simulink model "ME780_A3_Q3b"  (R2025b)
settings: Solver=FixedStepAuto  StartTime=0.0  StopTime=12  FixedStep=0.0005  RelTol=1e-3
libraries: Solver_SF x1, slpidlib x1
settings Model: Creator=r3anjum  LastModifiedBy=r3anjum

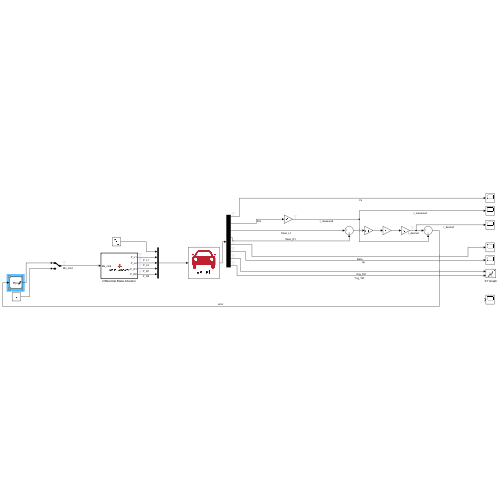
[thumbnail: Simulink's stored preview of the top-level diagram]
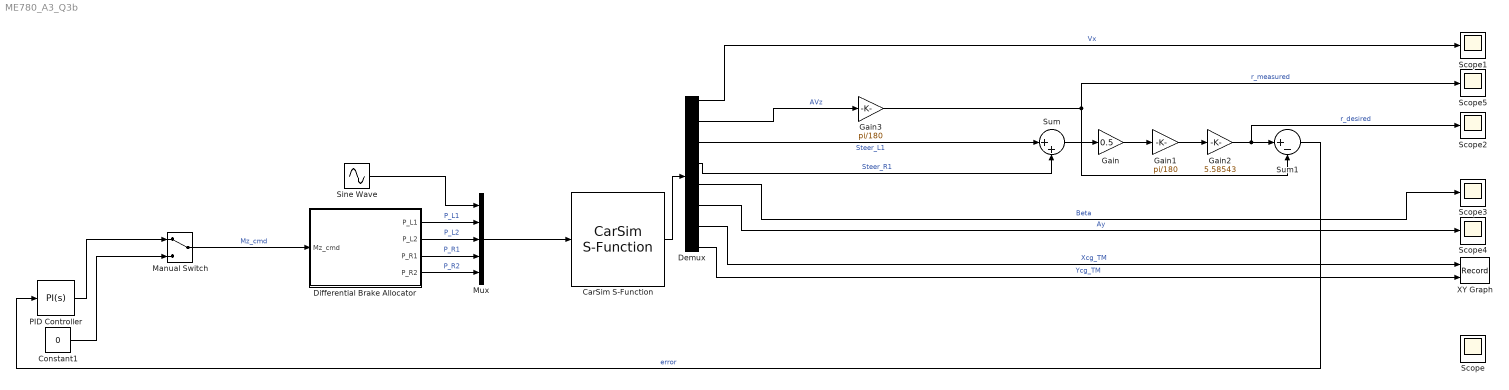
== system ME780_A3_Q3b ==
  CarSim S-Function : Solver_SF/CarSim S-Function  Priority=1  SIMFILE=simfile.sim  Run_RTs=off  vs_state_ind=Run  StopMode_ind=Vehicle Model
  Constant1 : Constant  Value=0
  Demux : Demux  Outputs=8
  Differential Brake Allocator : MATLAB Function  TreatAsAtomicUnit=on
  Gain : Gain  Gain=0.5
  Gain1 : Gain  Gain=pi/180
  Gain2 : Gain  Gain=5.58543
  Gain3 : Gain  Gain=pi/180
  Manual Switch : ManualSwitch
  Mux : Mux  Inputs=5
  PID Controller : slpidlib/PID Controller  Controller=PI  Form=Parallel  TimeDomain=Continuous-time  UseExternalTs=off  SampleTime=-1  IntegratorMethod=Forward Euler  FilterMethod=Forward Euler  ControllerParametersSource=internal  P=28835.61  I=57671.23  UseKiTs=off  D=0  UseExternalDerivativeSource=off  N=100  UseFilter=on  TunerSelectOption=Transfer Function Based (PID Tuner App)  InitialConditionSource=internal  InitialConditionForIntegrator=0  InitialConditionForFilter=0  DifferentiatorICPrevScaledInput=0  ExternalReset=none  TrackingMode=off  Kt=1  LimitOutput=on  SatLimitsSource=internal  UpperSaturationLimit=2800  LowerSaturationLimit=-2800  LinearizeAsGain=on  AntiWindupMode=clamping  Kb=1  LimitIntegrator=off  UpperIntegratorSaturationLimit=inf  LowerIntegratorSaturationLimit=-inf  POutMin=[]  POutMax=[]  IOutMin=[]  IOutMax=[]  DOutMin=[]  DOutMax=[]  NOutMin=[]  NOutMax=[]  SumOutMin=[]  SumOutMax=[]  SaturationOutMin=[]  SaturationOutMax=[]  PParamMin=[]  PParamMax=[]  IParamMin=[]  IParamMax=[]  DParamMin=[]  DParamMax=[]  NParamMin=[]  NParamMax=[]  KbParamMin=[]  KbParamMax=[]  KtParamMin=[]  KtParamMax=[]  KbOutMin=[]  KbOutMax=[]  KtOutMin=[]  KtOutMax=[]  IntegratorOutMin=[]  IntegratorOutMax=[]  FilterOutMin=[]  FilterOutMax=[]  SumI1OutMin=[]  SumI1OutMax=[]  SumI2OutMin=[]  SumI2OutMax=[]  SumI3OutMin=[]  SumI3OutMax=[]  SumI4OutMin=[]  SumI4OutMax=[]  SumDOutMin=[]  SumDOutMax=[]  DifferentiatorOutMin=[]  DifferentiatorOutMax=[]  FilterDiffOutCoefMin=[]  FilterDiffOutCoefMax=[]  ReciprocalOutMin=[]  ReciprocalOutMax=[]  SumDenOutMin=[]  SumDenOutMax=[]  SumNumOutMin=[]  SumNumOutMax=[]  DivideOutMin=[]  DivideOutMax=[]  UdiffTsProdOutMin=[]  UdiffTsProdOutMax=[]  NTsProdOutMin=[]  NTsProdOutMax=[]  UintegralTsProdOutMin=[]  UintegralTsProdOutMax=[]  UngainTsProdOutMin=[]  UngainTsProdOutMax=[]  ClampingZeroOutDataTypeStr=Inherit: Inherit via back propagation  ClampingZeroOutMin=[]  ClampingZeroOutMax=[]  FilterDenConstantOutDataTypeStr=Inherit: Inherit via back propagation  FilterDenConstantOutMin=[]  FilterDenConstantOutMax=[]  PCopyOutDataTypeStr=Inherit: Inherit via back propagation  PCopyOutMin=[]  PCopyOutMax=[]  NCopyOutDataTypeStr=Inherit: Inherit via back propagation  NCopyOutMin=[]  NCopyOutMax=[]  IntegratorContinuousStateAttributes=''  IntegratorStateMustResolveToSignalObject=off  IntegratorRTWStateStorageClass=Auto  FilterContinuousStateAttributes=''  FilterStateMustResolveToSignalObject=off  FilterRTWStateStorageClass=Auto  ParallelPVariant=InternalParameters  IdealPVariant=Disabled  IVariant=InternalParameters  DVariant=Disabled  IntegratorVariant=Continuous  SatVariant=Enabled  AWVariant=ContClampingParallel  PCopyVariant=Disabled  TRVariant=Disabled  FdbkBlocksVariant=Forward  IdealPFdbkVariant=Disabled  SatFdbkVariant=Disabled  DerivativeFilterVariant=Disabled  NVariant=Disabled  NCopyVariant=Disabled_SignalSpec  FilterICVariant=Disabled  IntegratorICVariant=InternalICs  ExternalResetVariant=Disabled  TRSumVariant=Passthrough  SumFdbkVariant=Disabled  SumVariant=Sum_PI  TsampFilterVariant=InternalTs  TsampNgainVariant=Passthrough  TsampIntegralVariant=Disabled_SignalSpec  ExternalSaturationOutDataTypeStr=Inherit: Same as second input  DerivativeSourceVariant=Disabled  PreIntVariant=InternalPreInt
  Scope{,1..5} (6 alike) : Scope
      Scope1 settings: ActiveDisplayYMinimum=-1  ActiveDisplayYMaximum=1
      Scope2 settings: DataLoggingVariableName=ScopeData2
      Scope3 settings: DataLoggingVariableName=ScopeData3
      Scope4 settings: DataLoggingVariableName=ScopeData4
      Scope5 settings: DataLoggingVariableName=ScopeData5
  Sine Wave : Sin  Amplitude=90  Frequency=pi/2  SampleTime=0
  Sum : Sum  Inputs=|++
  Sum1 : Sum  Inputs=|+-
  XY Graph : Record  NumPorts=2.0  FileSettingsInternal="{\"entries\":[{\"content\":{\"excelSettings\":{\"content\":{},\"type\":\"Streamout.ExcelSettings\"},\"parquetSettings\":{\"content\":{},\"type\":\"Streamout.ParquetSettings\"}},\"type\":\"Streamout.FileSettingStorage\",\"uuid\":\"\"}],\"packageUris\":[\"http:\\/\\/schema.mathworks.com\\/mf0\\/streamout_blocks\\/R2020a\"],\"version\":\"1.0\"}"  FrameSettings=[0, 0]  Layout=[1 1]  SignalsInternal="{\"entries\":[{\"content\":{},\"type\":\"RecordBlkView.InputSignals\",\"uuid\":\"\"}],\"packageUris\":[\"http:\\/\\/schema.mathworks.com\\/mf0\\/streamout_blocks\\/R2020a\"],\"version\":\"1.0\"}"  VisualizationBindings="{\"xyplotplugin\":{\"info\":[{\"series\":[],\"subplotID\":1}]}}"  CompatibilityTag=XY
  wires:
  Mux/1 -> CarSim S-Function/1
  Sine Wave/1 -> Mux/1
  CarSim S-Function/1 -> Demux/1
  Demux/1 -> Scope1/1  "Vx"
  Demux/2 -> Gain3/1  "AVz"
  Demux/3 -> Sum/1  "Steer_L1"
  Demux/4 -> Sum/2  "Steer_R1"
  Sum/1 -> Gain/1
  Gain/1 -> Gain1/1
  Gain1/1 -> Gain2/1
  Gain3/1 -> Sum1/2, Scope5/1  "r_measured"
  Gain2/1 -> Scope2/1, Sum1/1  "r_desired"
  PID Controller/1 -> Manual Switch/1
  Constant1/1 -> Manual Switch/2
  Sum1/1 -> PID Controller/1  "error"
  Demux/5 -> Scope3/1  "Beta"
  Demux/6 -> Scope4/1  "Ay"
  Demux/7 -> XY Graph/1  "Xcg_TM"
  Demux/8 -> XY Graph/2  "Ycg_TM"
  Manual Switch/1 -> Differential Brake Allocator/1(Mz_cmd)  "Mz_cmd"
  Differential Brake Allocator/1(P_L1) -> Mux/2  "P_L1"
  Differential Brake Allocator/2(P_L2) -> Mux/3  "P_L2"
  Differential Brake Allocator/3(P_R1) -> Mux/4  "P_R1"
  Differential Brake Allocator/4(P_R2) -> Mux/5  "P_R2"

== matlab function ME780_A3_Q3b/Differential Brake Allocator ==
  data: Mz_cmd input; P_L1 output; P_L2 output; P_R1 output; P_R2 output
function [P_L1, P_L2, P_R1, P_R2] = brake_allocator(Mz_cmd)
% Convert desired corrective yaw moment [N*m]
% into individual wheel brake pressures [MPa].

% Vehicle parameters
tf = 1.575;       % Front track width [m]
tr = 1.575;       % Rear track width [m]
Re = 0.393;       % Effective tire rolling radius [m]

% Front/rear corrective-moment allocation
lambda_f = 0.60;
lambda_r = 0.40;

% CarSim brake torque/pressure coefficients
Kbf = 350;        % Front brake coefficient [N*m/MPa]
Kbr = 150;        % Rear brake coefficient [N*m/MPa]

% Safety saturation on requested yaw moment
Mz = min(max(Mz_cmd, -2800), 2800);

% Required brake-pressure magnitudes
Pf = (2*Re*lambda_f/(tf*Kbf))*abs(Mz);
Pr = (2*Re*lambda_r/(tr*Kbr))*abs(Mz);

% Initialize all brake pressures to zero
P_L1 = 0;
P_L2 = 0;
P_R1 = 0;
P_R2 = 0;

% Initial left/right sign assumption
if Mz > 0
    % Positive requested yaw moment:
    % apply braking on the left side
    P_L1 = Pf;
    P_L2 = Pr;

elseif Mz < 0
    % Negative requested yaw moment:
    % apply braking on the right side
    P_R1 = Pf;
    P_R2 = Pr;
end

end
